simulink model "zajecia678910"  (R2022b)
settings: Solver=VariableStepAuto  StartTime=0  StopTime=t_simulation  MaxStep=0.1  RelTol=1e-3
values from neighbouring files (symbols this model uses):
  Cvp = cp * rop * Vp    (= 90000)    [zajecia678910matlab.m]
  Cvw = cp * rop * Vw    (= 150000)    [zajecia678910matlab.m]
  dTzad = 5    [zajecia678910matlab.m]
  dTzew = 0    [zajecia678910matlab.m]
  K = 0.003    [zajecia678910matlab.m]
  Kcp = (qgN*a*(TwewN-TpN))/((TwewN * (1 + a) - TzewN - a*TpN)  * (TpN - TzewN))    (= 19.6078431373)    [zajecia678910matlab.m]
  Kcw = qgN/(TwewN * (1 + a) - TzewN - a * TpN)    (= 235.294117647)    [zajecia678910matlab.m]
  Kcwp = a*Kcw    (= 58.8235294118)    [zajecia678910matlab.m]
  Ki = 1/Ti    (= 0.000556111667223)    [zajecia678910matlab.m]
  KiTunerModel = 1.4462    [zajecia678910matlab.m]
  KiTunerObjekt = 0.086692    [zajecia678910matlab.m]
  Kp = (0.9*TTp)/(K0Tp*T0Tp)    (= 763.333333333)    [zajecia678910matlab.m]
  KpTunerModel = 486.9693    [zajecia678910matlab.m]
  KpTunerObjekt = 584.5609    [zajecia678910matlab.m]
  qg0 = Twew0*(Kcw+Kcwp)-Tp0*Kcwp-Kcw*((Tp0*(Kcp+Kcwp)-Twew0*Kcwp)/Kcp)    (= 10000)    [zajecia678910matlab.m]
  t0 = 5000    [zajecia678910matlab.m]
  T0TpDP = 690    [zajecia678910matlab.m]
  Ti = 3.33*T0Tp    (= 1798.2)    [zajecia678910matlab.m]
  Tp0 = ((Kcw + Kcwp)*Kcp*Tzew0 + Kcwp*(qg0 + Kcw*Tzew0))/(Kcw*(Kcwp + Kcp) + Kcwp*Kcp)    (= 10)    [zajecia678910matlab.m]
  Twew0 = (qg0*(Kcwp + Kcp) + Tzew0*(Kcw*Kcwp + Kcw * Kcp + Kcwp * Kcp))/(Kcw*(Kcwp + Kcp) + Kcwp * Kcp)    (= 20)    [zajecia678910matlab.m]
  Tzad = TpN    (= 10)    [zajecia678910matlab.m]
  Tzew0 = TzewN    (= -20)    [zajecia678910matlab.m]
undefined symbols (not defined in the file or in its folder): qg0Model
libraries: slpidlib x2
settings Model: Creator=huber  LastModifiedBy=huber
settings DataIOCC: SaveFormat=StructureWithTime  ReturnWorkspaceOutputs=off
settings OptimizationCC: BlockReduction=off  BufferReuse=off
settings DebuggingCC: AlgebraicLoopMsg=none

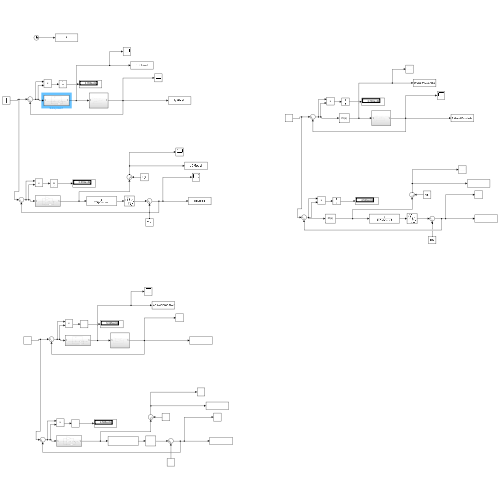
[thumbnail: Simulink's stored preview of the top-level diagram]
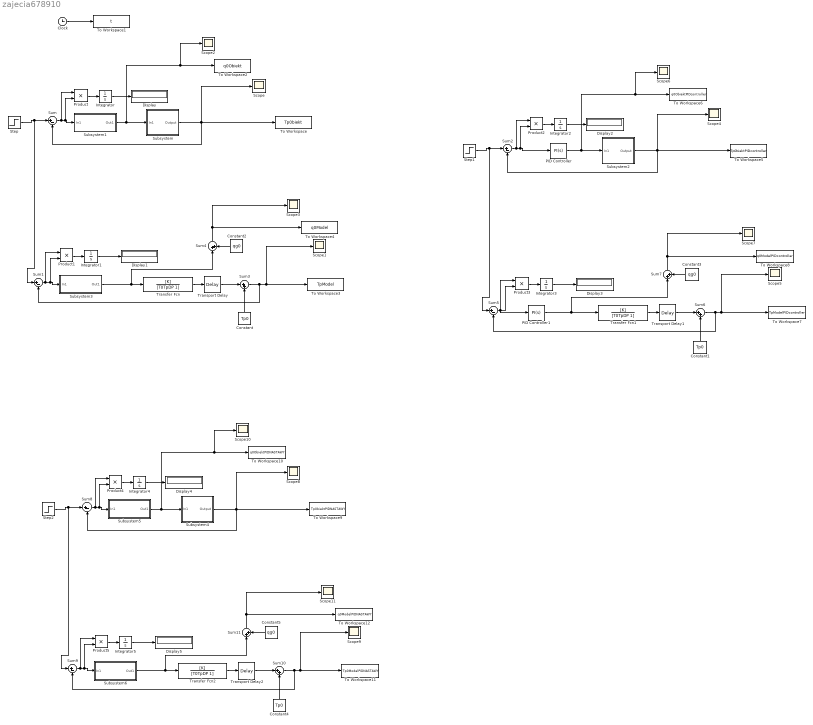
== system zajecia678910 ==
  Clock : Clock
  Constant : Constant  Value=Tp0
  Constant1 : Constant  Value=Tp0
  Constant2 : Constant  Value=qg0
  Constant3 : Constant  Value=qg0
  Constant4 : Constant  Value=Tp0
  Constant5 : Constant  Value=qg0
  Display{,1..5} (6 alike) : Display
  Integrator{,1..5} (6 alike) : Integrator
  PID Controller : slpidlib/PID Controller  Controller=PI  Form=Parallel  TimeDomain=Continuous-time  UseExternalTs=off  SampleTime=-1  IntegratorMethod=Forward Euler  FilterMethod=Forward Euler  ControllerParametersSource=internal  P=KpTunerObjekt  I=KiTunerObjekt  UseKiTs=off  D=0  N=100  UseFilter=on  TunerSelectOption=Transfer Function Based (PID Tuner App)  InitialConditionSource=internal  InitialConditionForIntegrator=qg0Model  InitialConditionForFilter=0  DifferentiatorICPrevScaledInput=0  ExternalReset=none  TrackingMode=off  Kt=1  LimitOutput=off  SatLimitsSource=internal  UpperSaturationLimit=inf  LowerSaturationLimit=-inf  LinearizeAsGain=on  AntiWindupMode=none  Kb=1  LimitIntegrator=off  UpperIntegratorSaturationLimit=inf  LowerIntegratorSaturationLimit=-inf  POutMin=[]  POutMax=[]  IOutMin=[]  IOutMax=[]  DOutMin=[]  DOutMax=[]  NOutMin=[]  NOutMax=[]  SumOutMin=[]  SumOutMax=[]  SaturationOutMin=[]  SaturationOutMax=[]  PParamMin=[]  PParamMax=[]  IParamMin=[]  IParamMax=[]  DParamMin=[]  DParamMax=[]  NParamMin=[]  NParamMax=[]  KbParamMin=[]  KbParamMax=[]  KtParamMin=[]  KtParamMax=[]  KbOutMin=[]  KbOutMax=[]  KtOutMin=[]  KtOutMax=[]  IntegratorOutMin=[]  IntegratorOutMax=[]  FilterOutMin=[]  FilterOutMax=[]  SumI1OutMin=[]  SumI1OutMax=[]  SumI2OutMin=[]  SumI2OutMax=[]  SumI3OutMin=[]  SumI3OutMax=[]  SumI4OutMin=[]  SumI4OutMax=[]  SumDOutMin=[]  SumDOutMax=[]  DifferentiatorOutMin=[]  DifferentiatorOutMax=[]  FilterDiffOutCoefMin=[]  FilterDiffOutCoefMax=[]  ReciprocalOutMin=[]  ReciprocalOutMax=[]  SumDenOutMin=[]  SumDenOutMax=[]  SumNumOutMin=[]  SumNumOutMax=[]  DivideOutMin=[]  DivideOutMax=[]  UdiffTsProdOutMin=[]  UdiffTsProdOutMax=[]  NTsProdOutMin=[]  NTsProdOutMax=[]  UintegralTsProdOutMin=[]  UintegralTsProdOutMax=[]  UngainTsProdOutMin=[]  UngainTsProdOutMax=[]  ClampingZeroOutDataTypeStr=Inherit: Inherit via back propagation  ClampingZeroOutMin=[]  ClampingZeroOutMax=[]  FilterDenConstantOutDataTypeStr=Inherit: Inherit via back propagation  FilterDenConstantOutMin=[]  FilterDenConstantOutMax=[]  PCopyOutDataTypeStr=Inherit: Inherit via back propagation  PCopyOutMin=[]  PCopyOutMax=[]  NCopyOutDataTypeStr=Inherit: Inherit via back propagation  NCopyOutMin=[]  NCopyOutMax=[]  IntegratorContinuousStateAttributes=''  IntegratorStateMustResolveToSignalObject=off  IntegratorRTWStateStorageClass=Auto  FilterContinuousStateAttributes=''  FilterStateMustResolveToSignalObject=off  FilterRTWStateStorageClass=Auto  ParallelPVariant=InternalParameters  IdealPVariant=Disabled  IVariant=InternalParameters  DVariant=InternalParameters  IntegratorVariant=Continuous  SatVariant=Disabled  AWVariant=Passthrough  PCopyVariant=Disabled  TRVariant=Disabled  FdbkBlocksVariant=Forward  IdealPFdbkVariant=Disabled  SatFdbkVariant=Disabled  DerivativeFilterVariant=ContFilter  NVariant=InternalParameters  NCopyVariant=Disabled  FilterICVariant=InternalICsFilter  IntegratorICVariant=InternalICs  ExternalResetVariant=Disabled  TRSumVariant=Passthrough  SumFdbkVariant=Disabled  SumVariant=Sum_PID  TsampFilterVariant=InternalTs  TsampNgainVariant=Passthrough  TsampIntegralVariant=Passthrough  ExternalSaturationOutDataTypeStr=Inherit: Same as second input
  PID Controller1 : slpidlib/PID Controller  Controller=PI  Form=Parallel  TimeDomain=Continuous-time  UseExternalTs=off  SampleTime=-1  IntegratorMethod=Forward Euler  FilterMethod=Forward Euler  ControllerParametersSource=internal  P=KpTunerModel  I=KiTunerModel  UseKiTs=off  D=0  N=100  UseFilter=on  TunerSelectOption=Transfer Function Based (PID Tuner App)  InitialConditionSource=internal  InitialConditionForIntegrator=0  InitialConditionForFilter=0  DifferentiatorICPrevScaledInput=0  ExternalReset=none  TrackingMode=off  Kt=1  LimitOutput=off  SatLimitsSource=internal  UpperSaturationLimit=inf  LowerSaturationLimit=-inf  LinearizeAsGain=on  AntiWindupMode=none  Kb=1  LimitIntegrator=off  UpperIntegratorSaturationLimit=inf  LowerIntegratorSaturationLimit=-inf  POutMin=[]  POutMax=[]  IOutMin=[]  IOutMax=[]  DOutMin=[]  DOutMax=[]  NOutMin=[]  NOutMax=[]  SumOutMin=[]  SumOutMax=[]  SaturationOutMin=[]  SaturationOutMax=[]  PParamMin=[]  PParamMax=[]  IParamMin=[]  IParamMax=[]  DParamMin=[]  DParamMax=[]  NParamMin=[]  NParamMax=[]  KbParamMin=[]  KbParamMax=[]  KtParamMin=[]  KtParamMax=[]  KbOutMin=[]  KbOutMax=[]  KtOutMin=[]  KtOutMax=[]  IntegratorOutMin=[]  IntegratorOutMax=[]  FilterOutMin=[]  FilterOutMax=[]  SumI1OutMin=[]  SumI1OutMax=[]  SumI2OutMin=[]  SumI2OutMax=[]  SumI3OutMin=[]  SumI3OutMax=[]  SumI4OutMin=[]  SumI4OutMax=[]  SumDOutMin=[]  SumDOutMax=[]  DifferentiatorOutMin=[]  DifferentiatorOutMax=[]  FilterDiffOutCoefMin=[]  FilterDiffOutCoefMax=[]  ReciprocalOutMin=[]  ReciprocalOutMax=[]  SumDenOutMin=[]  SumDenOutMax=[]  SumNumOutMin=[]  SumNumOutMax=[]  DivideOutMin=[]  DivideOutMax=[]  UdiffTsProdOutMin=[]  UdiffTsProdOutMax=[]  NTsProdOutMin=[]  NTsProdOutMax=[]  UintegralTsProdOutMin=[]  UintegralTsProdOutMax=[]  UngainTsProdOutMin=[]  UngainTsProdOutMax=[]  ClampingZeroOutDataTypeStr=Inherit: Inherit via back propagation  ClampingZeroOutMin=[]  ClampingZeroOutMax=[]  FilterDenConstantOutDataTypeStr=Inherit: Inherit via back propagation  FilterDenConstantOutMin=[]  FilterDenConstantOutMax=[]  PCopyOutDataTypeStr=Inherit: Inherit via back propagation  PCopyOutMin=[]  PCopyOutMax=[]  NCopyOutDataTypeStr=Inherit: Inherit via back propagation  NCopyOutMin=[]  NCopyOutMax=[]  IntegratorContinuousStateAttributes=''  IntegratorStateMustResolveToSignalObject=off  IntegratorRTWStateStorageClass=Auto  FilterContinuousStateAttributes=''  FilterStateMustResolveToSignalObject=off  FilterRTWStateStorageClass=Auto  ParallelPVariant=InternalParameters  IdealPVariant=Disabled  IVariant=InternalParameters  DVariant=InternalParameters  IntegratorVariant=Continuous  SatVariant=Disabled  AWVariant=Passthrough  PCopyVariant=Disabled  TRVariant=Disabled  FdbkBlocksVariant=Forward  IdealPFdbkVariant=Disabled  SatFdbkVariant=Disabled  DerivativeFilterVariant=ContFilter  NVariant=InternalParameters  NCopyVariant=Disabled  FilterICVariant=InternalICsFilter  IntegratorICVariant=InternalICs  ExternalResetVariant=Disabled  TRSumVariant=Passthrough  SumFdbkVariant=Disabled  SumVariant=Sum_PID  TsampFilterVariant=InternalTs  TsampNgainVariant=Passthrough  TsampIntegralVariant=Passthrough  ExternalSaturationOutDataTypeStr=Inherit: Same as second input
  Product{,1..5} (6 alike) : Product
  Scope{,1..11} (12 alike) : Scope
  Step : Step  Time=t0  Before=1  After=Tzad + dTzad  SampleTime=0
  Step1 : Step  Time=t0  Before=1  After=Tzad + dTzad  SampleTime=0
  Step2 : Step  Time=t0  Before=1  After=Tzad + dTzad  SampleTime=0
  Subsystem : Subsystem
  Subsystem1 : Subsystem
  Subsystem2 : Subsystem
  Subsystem3 : Subsystem
  Subsystem4 : Subsystem
  Subsystem5 : Subsystem
  Subsystem6 : Subsystem
  Sum{,1..2,5,8..9} (6 alike) : Sum  Inputs=|+-
  Sum{3..4,6..7,10..11} (6 alike) : Sum  Inputs=|++
  To Workspace : ToWorkspace  VariableName=Tp0biekt  SampleTime=-1
  To Workspace1 : ToWorkspace  VariableName=t  SampleTime=-1
  To Workspace10 : ToWorkspace  VariableName=q0ObiektPIDNASTAWY  SampleTime=-1
  To Workspace11 : ToWorkspace  VariableName=Tp0ModelPIDNASTAWY  SampleTime=-1
  To Workspace12 : ToWorkspace  VariableName=q0ModelPIDNASTAWY  SampleTime=-1
  To Workspace2 : ToWorkspace  VariableName=q0Obiekt  SampleTime=-1
  To Workspace3 : ToWorkspace  VariableName=TpModel  SampleTime=-1
  To Workspace4 : ToWorkspace  VariableName=q0Model  SampleTime=-1
  To Workspace5 : ToWorkspace  VariableName=Tp0biektPIDcontroller  SampleTime=-1
  To Workspace6 : ToWorkspace  VariableName=q0ObiektPIDcontroller  SampleTime=-1
  To Workspace7 : ToWorkspace  VariableName=TpModelPIDcontroller  SampleTime=-1
  To Workspace8 : ToWorkspace  VariableName=q0ModelPIDcontroller  SampleTime=-1
  To Workspace9 : ToWorkspace  VariableName=Tp0biektPIDNASTAWY  SampleTime=-1
  Transfer Fcn : TransferFcn  Numerator=[K]  Denominator=[T0TpDP 1]
  Transfer Fcn1 : TransferFcn  Numerator=[K]  Denominator=[T0TpDP 1]
  Transfer Fcn2 : TransferFcn  Numerator=[K]  Denominator=[T0TpDP 1]
  Transport Delay : TransportDelay  DelayTime=86
  Transport Delay1 : TransportDelay  DelayTime=86
  Transport Delay2 : TransportDelay  DelayTime=86
  wires:
  Sum/1 -> Product/1, Product/2, Subsystem1/1(In1)
  Step/1 -> Sum1/1, Sum/1
  Clock/1 -> To Workspace1/1
  Subsystem/1(Output) -> To Workspace/1, Scope/1, Sum/2
  Subsystem1/1(Out1) -> Scope2/1, To Workspace2/1, Subsystem/1(In1)
  Subsystem3/1(Out1) -> Sum4/1, Transfer Fcn/1
  Sum1/1 -> Product1/1, Product1/2, Subsystem3/1(In1)
  Transfer Fcn/1 -> Transport Delay/1
  Transport Delay/1 -> Sum3/1
  Sum3/1 -> Sum1/2, Scope1/1, To Workspace3/1
  Integrator/1 -> Display/1
  Product/1 -> Integrator/1
  Product1/1 -> Integrator1/1
  Integrator1/1 -> Display1/1
  Constant/1 -> Sum3/2
  Sum4/1 -> To Workspace4/1, Scope3/1
  Constant2/1 -> Sum4/2
  Sum7/1 -> To Workspace8/1, Scope7/1
  Constant1/1 -> Sum6/2
  Subsystem2/1(Output) -> To Workspace5/1, Scope4/1, Sum2/2
  Sum2/1 -> Product2/1, PID Controller/1, Product2/2
  Integrator3/1 -> Display3/1
  Constant3/1 -> Sum7/2
  Product3/1 -> Integrator3/1
  Step1/1 -> Sum5/1, Sum2/1
  Product2/1 -> Integrator2/1
  Sum6/1 -> Sum5/2, Scope5/1, To Workspace7/1
  Transfer Fcn1/1 -> Transport Delay1/1
  Sum5/1 -> Product3/1, Product3/2, PID Controller1/1
  Integrator2/1 -> Display2/1
  Transport Delay1/1 -> Sum6/1
  PID Controller/1 -> Scope6/1, To Workspace6/1, Subsystem2/1(In1)
  PID Controller1/1 -> Sum7/1, Transfer Fcn1/1
  Sum11/1 -> To Workspace12/1, Scope11/1
  Constant4/1 -> Sum10/2
  Transfer Fcn2/1 -> Transport Delay2/1
  Sum8/1 -> Product4/1, Product4/2, Subsystem5/1(In1)
  Subsystem4/1(Output) -> To Workspace9/1, Scope8/1, Sum8/2
  Product4/1 -> Integrator4/1
  Subsystem5/1(Out1) -> Scope10/1, To Workspace10/1, Subsystem4/1(In1)
  Constant5/1 -> Sum11/2
  Transport Delay2/1 -> Sum10/1
  Integrator5/1 -> Display5/1
  Product5/1 -> Integrator5/1
  Integrator4/1 -> Display4/1
  Sum10/1 -> Sum9/2, Scope9/1, To Workspace11/1
  Sum9/1 -> Product5/1, Product5/2, Subsystem6/1(In1)
  Step2/1 -> Sum9/1, Sum8/1
  Subsystem6/1(Out1) -> Sum11/1, Transfer Fcn2/1

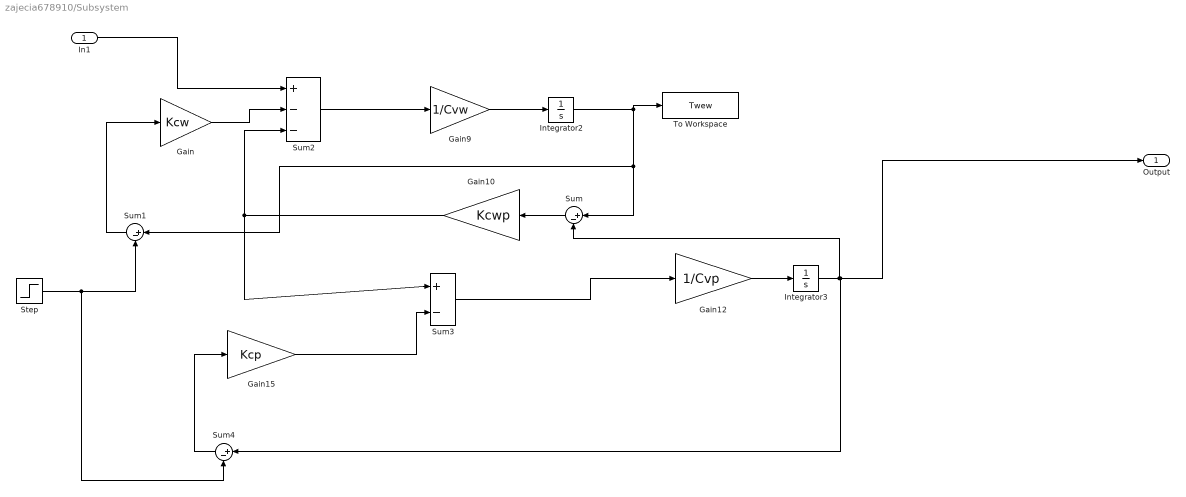
== system zajecia678910/Subsystem ==
  In1 : Inport
  Gain : Gain  Gain=Kcw
  Gain10 : Gain  Gain=Kcwp
  Gain12 : Gain  Gain=1/Cvp
  Gain15 : Gain  Gain=Kcp
  Gain9 : Gain  Gain=1/Cvw
  Integrator2 : Integrator  InitialCondition=Twew0
  Integrator3 : Integrator  InitialCondition=Tp0
  Step : Step  Time=t0  Before=Tzew0  After=Tzew0 + dTzew  SampleTime=0
  Sum{,1,3..4} (4 alike) : Sum  Inputs=|+-
  Sum2 : Sum  Inputs=+--
  To Workspace : ToWorkspace  VariableName=Twew  SampleTime=-1
  Output : Outport
  wires:
  Gain12/1 -> Integrator3/1
  Integrator2/1 -> To Workspace/1, Sum1/1, Sum/1
  Sum2/1 -> Gain9/1
  Gain9/1 -> Integrator2/1
  Gain10/1 -> Sum2/3, Sum3/1
  Integrator3/1 -> Output/1, Sum4/1, Sum/2
  Sum3/1 -> Gain12/1
  Gain15/1 -> Sum3/2
  In1/1 -> Sum2/1
  Step/1 -> Sum4/2, Sum1/2
  Gain/1 -> Sum2/2
  Sum1/1 -> Gain/1
  Sum/1 -> Gain10/1
  Sum4/1 -> Gain15/1

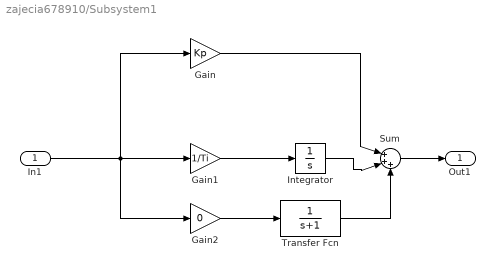
== system zajecia678910/Subsystem1 ==
  In1 : Inport
  Gain : Gain  Gain=Kp
  Gain1 : Gain  Gain=1/Ti
  Gain2 : Gain  Gain=0
  Integrator : Integrator  InitialCondition=qg0Model
  Sum : Sum  Inputs=|+++
  Transfer Fcn : TransferFcn  Denominator=[1 1]
  Out1 : Outport
  wires:
  In1/1 -> Gain2/1, Gain1/1, Gain/1
  Gain2/1 -> Transfer Fcn/1
  Gain/1 -> Sum/1
  Transfer Fcn/1 -> Sum/3
  Sum/1 -> Out1/1
  Gain1/1 -> Integrator/1
  Integrator/1 -> Sum/2

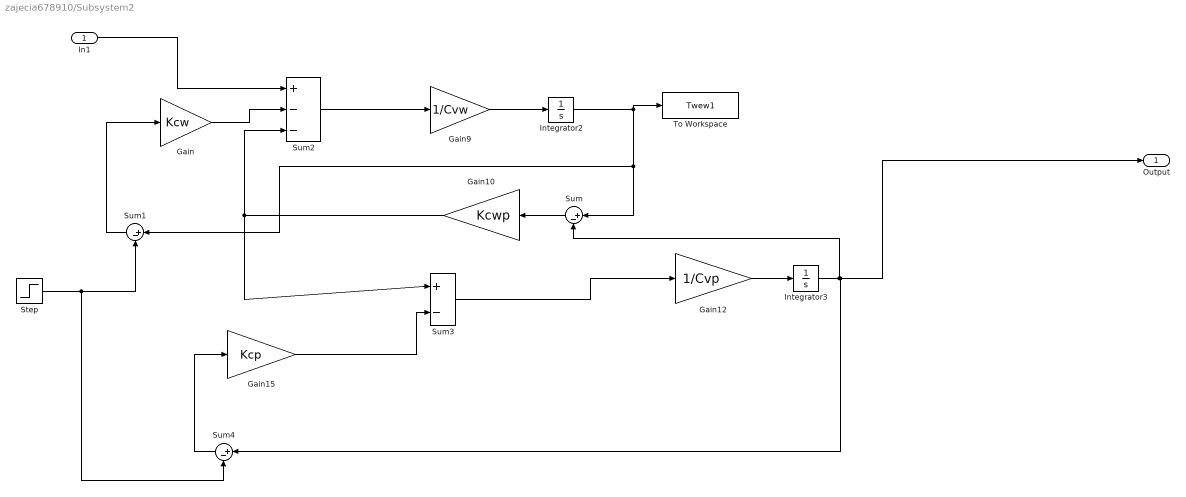
== system zajecia678910/Subsystem2 ==
  In1 : Inport
  Gain : Gain  Gain=Kcw
  Gain10 : Gain  Gain=Kcwp
  Gain12 : Gain  Gain=1/Cvp
  Gain15 : Gain  Gain=Kcp
  Gain9 : Gain  Gain=1/Cvw
  Integrator2 : Integrator  InitialCondition=Twew0
  Integrator3 : Integrator  InitialCondition=Tp0
  Step : Step  Time=t0  Before=Tzew0  After=Tzew0 + dTzew  SampleTime=0
  Sum{,1,3..4} (4 alike) : Sum  Inputs=|+-
  Sum2 : Sum  Inputs=+--
  To Workspace : ToWorkspace  VariableName=Twew1  SampleTime=-1
  Output : Outport
  wires:
  Gain12/1 -> Integrator3/1
  Integrator2/1 -> To Workspace/1, Sum1/1, Sum/1
  Sum2/1 -> Gain9/1
  Gain9/1 -> Integrator2/1
  Gain10/1 -> Sum2/3, Sum3/1
  Integrator3/1 -> Output/1, Sum4/1, Sum/2
  Sum3/1 -> Gain12/1
  Gain15/1 -> Sum3/2
  In1/1 -> Sum2/1
  Step/1 -> Sum4/2, Sum1/2
  Gain/1 -> Sum2/2
  Sum1/1 -> Gain/1
  Sum/1 -> Gain10/1
  Sum4/1 -> Gain15/1

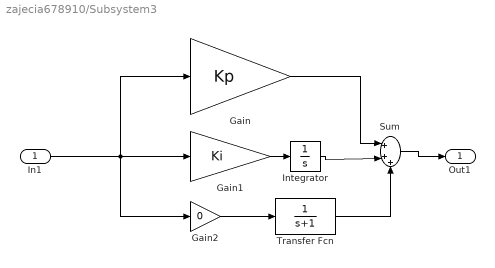
== system zajecia678910/Subsystem3 ==
  In1 : Inport
  Gain : Gain  Gain=Kp
  Gain1 : Gain  Gain=Ki
  Gain2 : Gain  Gain=0
  Integrator : Integrator
  Sum : Sum  Inputs=|+++
  Transfer Fcn : TransferFcn  Denominator=[1 1]
  Out1 : Outport
  wires:
  In1/1 -> Gain/1, Gain1/1, Gain2/1
  Gain/1 -> Sum/1
  Transfer Fcn/1 -> Sum/3
  Sum/1 -> Out1/1
  Gain2/1 -> Transfer Fcn/1
  Gain1/1 -> Integrator/1
  Integrator/1 -> Sum/2

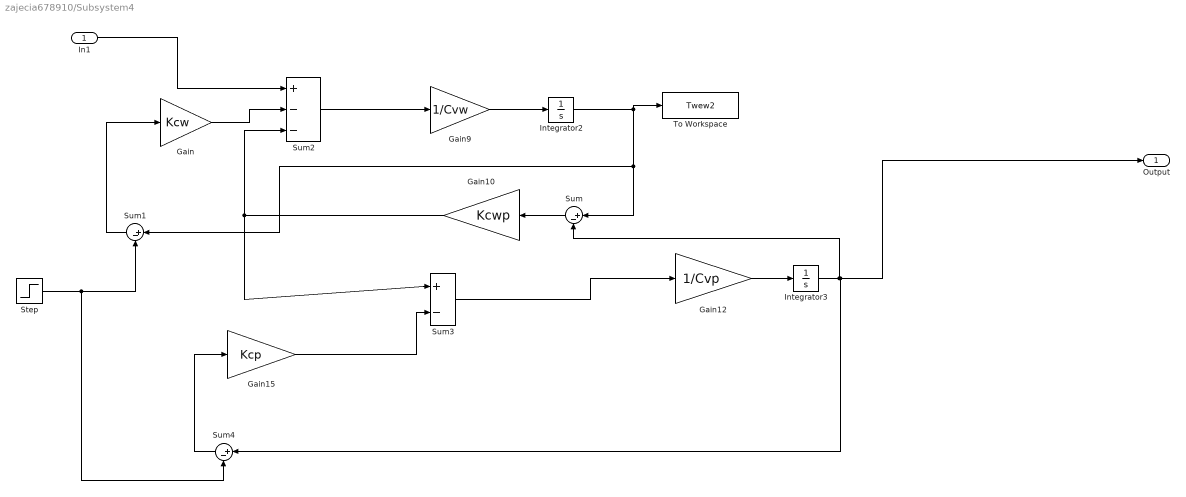
== system zajecia678910/Subsystem4 ==
  In1 : Inport
  Gain : Gain  Gain=Kcw
  Gain10 : Gain  Gain=Kcwp
  Gain12 : Gain  Gain=1/Cvp
  Gain15 : Gain  Gain=Kcp
  Gain9 : Gain  Gain=1/Cvw
  Integrator2 : Integrator  InitialCondition=Twew0
  Integrator3 : Integrator  InitialCondition=Tp0
  Step : Step  Time=t0  Before=Tzew0  After=Tzew0 + dTzew  SampleTime=0
  Sum{,1,3..4} (4 alike) : Sum  Inputs=|+-
  Sum2 : Sum  Inputs=+--
  To Workspace : ToWorkspace  VariableName=Twew2  SampleTime=-1
  Output : Outport
  wires:
  Gain12/1 -> Integrator3/1
  Integrator2/1 -> To Workspace/1, Sum1/1, Sum/1
  Sum2/1 -> Gain9/1
  Gain9/1 -> Integrator2/1
  Gain10/1 -> Sum2/3, Sum3/1
  Integrator3/1 -> Output/1, Sum4/1, Sum/2
  Sum3/1 -> Gain12/1
  Gain15/1 -> Sum3/2
  In1/1 -> Sum2/1
  Step/1 -> Sum4/2, Sum1/2
  Gain/1 -> Sum2/2
  Sum1/1 -> Gain/1
  Sum/1 -> Gain10/1
  Sum4/1 -> Gain15/1

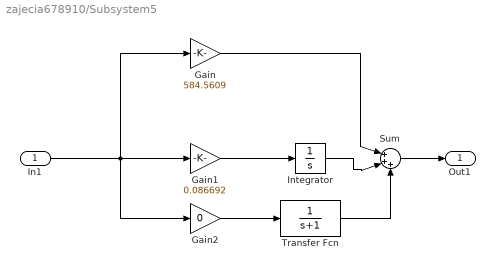
== system zajecia678910/Subsystem5 ==
  In1 : Inport
  Gain : Gain  Gain=584.5609
  Gain1 : Gain  Gain=0.086692
  Gain2 : Gain  Gain=0
  Integrator : Integrator  InitialCondition=qg0Model
  Sum : Sum  Inputs=|+++
  Transfer Fcn : TransferFcn  Denominator=[1 1]
  Out1 : Outport
  wires:
  In1/1 -> Gain2/1, Gain1/1, Gain/1
  Gain2/1 -> Transfer Fcn/1
  Gain/1 -> Sum/1
  Transfer Fcn/1 -> Sum/3
  Sum/1 -> Out1/1
  Gain1/1 -> Integrator/1
  Integrator/1 -> Sum/2

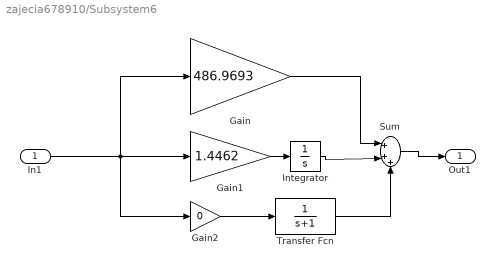
== system zajecia678910/Subsystem6 ==
  In1 : Inport
  Gain : Gain  Gain=486.9693
  Gain1 : Gain  Gain=1.4462
  Gain2 : Gain  Gain=0
  Integrator : Integrator
  Sum : Sum  Inputs=|+++
  Transfer Fcn : TransferFcn  Denominator=[1 1]
  Out1 : Outport
  wires:
  In1/1 -> Gain/1, Gain1/1, Gain2/1
  Gain/1 -> Sum/1
  Transfer Fcn/1 -> Sum/3
  Sum/1 -> Out1/1
  Gain2/1 -> Transfer Fcn/1
  Gain1/1 -> Integrator/1
  Integrator/1 -> Sum/2
